simulink model "Std_Test_Signal"  (R2024b)
settings: Solver=FixedStepAuto  StartTime=0.0  StopTime=10.0  FixedStep=0.001  RelTol=1e-3
libraries: simulink x1
settings Model: Creator=abdal  LastModifiedBy=abdal

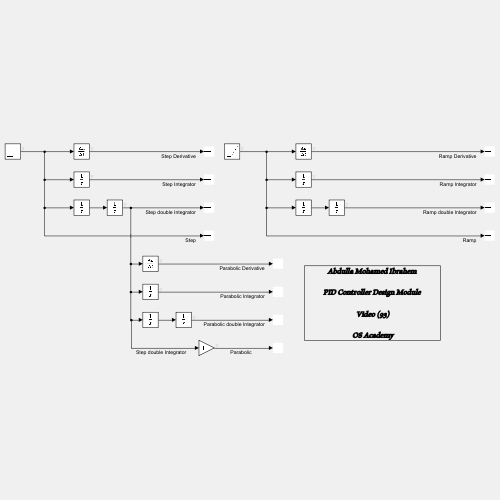
[thumbnail: Simulink's stored preview of the top-level diagram]
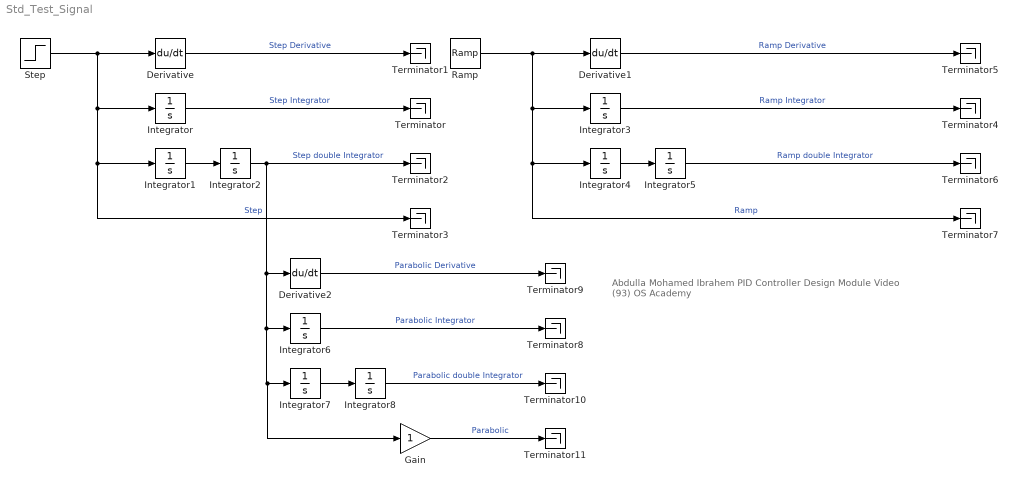
== system Std_Test_Signal ==
  note: Abdulla Mohamed Ibrahem
      | PID Controller Design Module
      | Video (93)
      | OS Academy
  Derivative : Derivative
  Derivative1 : Derivative
  Derivative2 : Derivative
  Gain : Gain
  Integrator{,1..8} (9 alike) : Integrator
  Ramp : simulink/Sources/Ramp  slope=3  start=3  InitialOutput=2
  Step : Step  Time=3  After=5  SampleTime=0
  Terminator{,1..11} (12 alike) : Terminator
  wires:
  Integrator1/1 -> Integrator2/1
  Integrator/1 -> Terminator/1  "Step Integrator"
  Derivative/1 -> Terminator1/1  "Step Derivative"
  Integrator2/1 -> Terminator2/1, Gain/1, Integrator7/1, Integrator6/1, Derivative2/1  "Step double Integrator"
  Integrator5/1 -> Terminator6/1  "Ramp double Integrator"
  Derivative1/1 -> Terminator5/1  "Ramp Derivative"
  Integrator3/1 -> Terminator4/1  "Ramp Integrator"
  Integrator4/1 -> Integrator5/1
  Ramp/1 -> Derivative1/1, Integrator3/1, Integrator4/1, Terminator7/1  "Ramp"
  Integrator8/1 -> Terminator10/1  "Parabolic double Integrator"
  Derivative2/1 -> Terminator9/1  "Parabolic Derivative"
  Integrator6/1 -> Terminator8/1  "Parabolic Integrator"
  Integrator7/1 -> Integrator8/1
  Step/1 -> Terminator3/1, Integrator1/1, Integrator/1, Derivative/1  "Step"
  Gain/1 -> Terminator11/1  "Parabolic"
